simulink model "acc_integrated_model"  (R2024b)
settings: Solver=FixedStepDiscrete  StartTime=0.0  StopTime=inf  FixedStep=0.05  RelTol=1e-3
model workspace (MAT data in the model file):
  command_bp = [0 1 2 3 4 5 6 7]
  control_enabled_table = [1  1  1  1  1  1  0  0; 0  1  1  0  0  0  0  0; 0  1  0  0  0  0  0  0; 0  0  0  0  0  0  0  0]
  decision_raw_table = [-1  1  2  3  4  7  8  8; 8  5  6  8  8  8  8  8; 8  5  8  8  8  8  8  8; 8  8  8  8  8  8  8  8]
  decision_table = [-1  1  2  3  4  7  8  8; 8  5  6  8  8  8  8  8; 8  5  8  8  8  8  8  8; 8  8  8  8  8  8  8  8]
  next_state_table = [0  0  0  0  0  0  1  1; 1  0  0  1  1  1  1  1; 2  0  2  2  2  2  2  2; 3  3  3  3  3  3  3  3]
  side_effect_table = [0  0  0  0  0  0  0  0; 0  0  0  0  0  0  0  0; 0  1  0  0  0  0  0  0; 0  0  0  0  0  0  0  0]
  state_bp = [0 1 2 3]
undefined symbols (not defined in the file or in its folder): dspblkCoreblockFVToolHelper, f, gcbh
libraries: simulink x3, instrumentlib x2, sldvlib x1
settings Model: Creator=aiden  LastModifiedBy=aiden
settings DataIOCC: SaveOutput=off  SaveTime=off

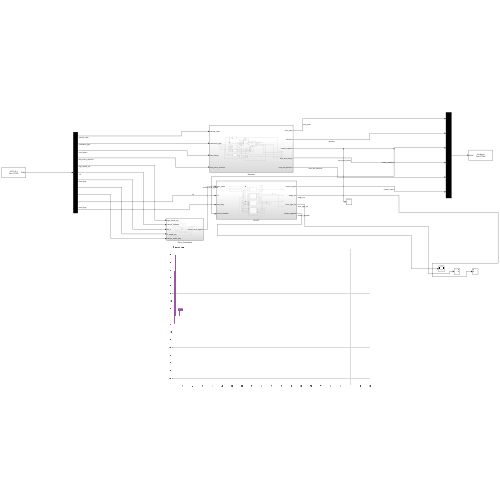
[thumbnail: Simulink's stored preview of the top-level diagram]
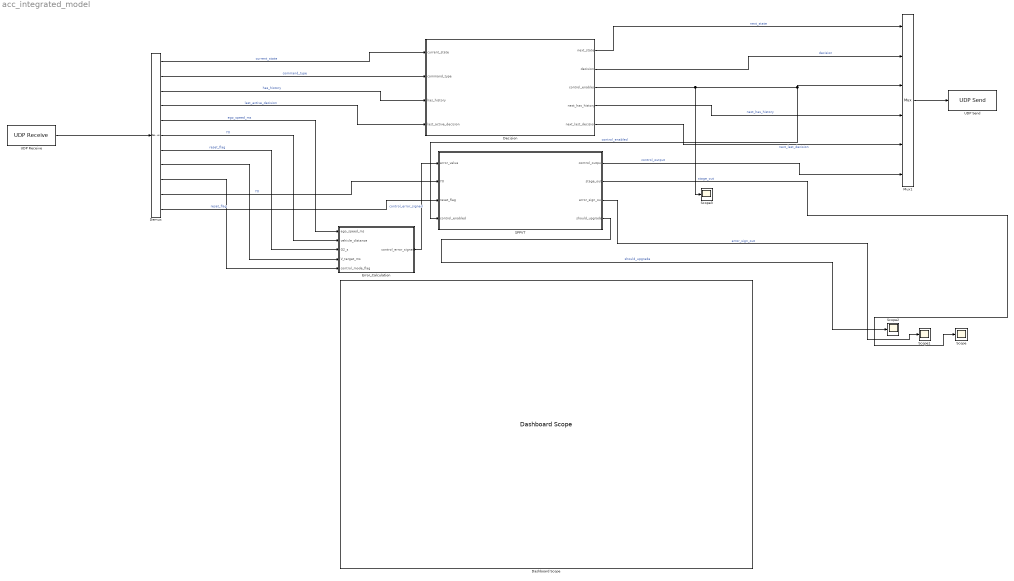
== system acc_integrated_model ==
  Dashboard Scope : DashboardScope  UpdateMode=Scroll
  Decision : Subsystem
  Demux : Demux  Outputs=11
  Error_Calculation : Subsystem
  Mux1 : Mux  Inputs=6
  SPPVT : Subsystem
  Scope{,1..3} (4 alike) : Scope
  UDP Receive : instrumentlib/UDP Receive  LocalAddress=127.0.0.1  LocalPort=27000  EnablePortSharing=off  Host=localhost  Port=9090  GetLatestData=on  DataSize=[ 11, 1 ]  DataType=double  ASCIIFormatting=%f,  Terminator=LF  CustomTerminator=10  ByteOrder=little-endian  EnableBlockingMode=on  Timeout=20  SampleTime=-1  SimulateUsing=Interpreted execution
  UDP Send : instrumentlib/UDP Send  Host=localhost  Port=27001  LocalAddress=0.0.0.0  LocalPort=27001  EnablePortSharing=on  OutputDatagramPacketSize=512  ByteOrder=little-endian  EnableBlockingMode=off  SimulateUsing=Interpreted execution
  wires:
  UDP Receive/1 -> Demux/1
  Demux/1 -> Decision/1(current_state)  "current_state"
  Demux/2 -> Decision/2(command_type)  "command_type"
  Demux/3 -> Decision/3(has_history)  "has_history"
  Demux/4 -> Decision/4(last_active_decision)  "last_active_decision"
  Error_Calculation/1(control_error_signed) -> SPPVT/1(error_value)  "control_error_signed"
  Demux/10 -> SPPVT/2(Y0)  "Y0"
  Demux/11 -> SPPVT/3(reset_flag)  "reset_flag"
  Decision/1(next_state) -> Mux1/1  "next_state"
  Decision/2(decision) -> Mux1/2  "decision"
  Decision/3(control_enabled) -> Scope3/1, Mux1/3, SPPVT/4(control_enabled)  "control_enabled"
  Decision/4(next_has_history) -> Mux1/4  "next_has_history"
  Decision/5(next_last_decision) -> Mux1/5  "next_last_decision"
  SPPVT/1(control_output) -> Mux1/6  "control_output"
  Mux1/1 -> UDP Send/1
  SPPVT/2(stage_out) -> Scope/1  "stage_out"
  SPPVT/3(error_sign_out) -> Scope1/1  "error_sign_out"
  SPPVT/4(should_upgrade) -> Scope2/1  "should_upgrade"
  Demux/5 -> Error_Calculation/1(ego_speed_ms)  "ego_speed_ms"
  Demux/6 -> Error_Calculation/2(vehicle_distance)  "Y0"
  Demux/7 -> Error_Calculation/3(G2_s)  "reset_flag"
  Demux/8 -> Error_Calculation/4(V_target_ms)
  Demux/9 -> Error_Calculation/5(control_mode_flag)

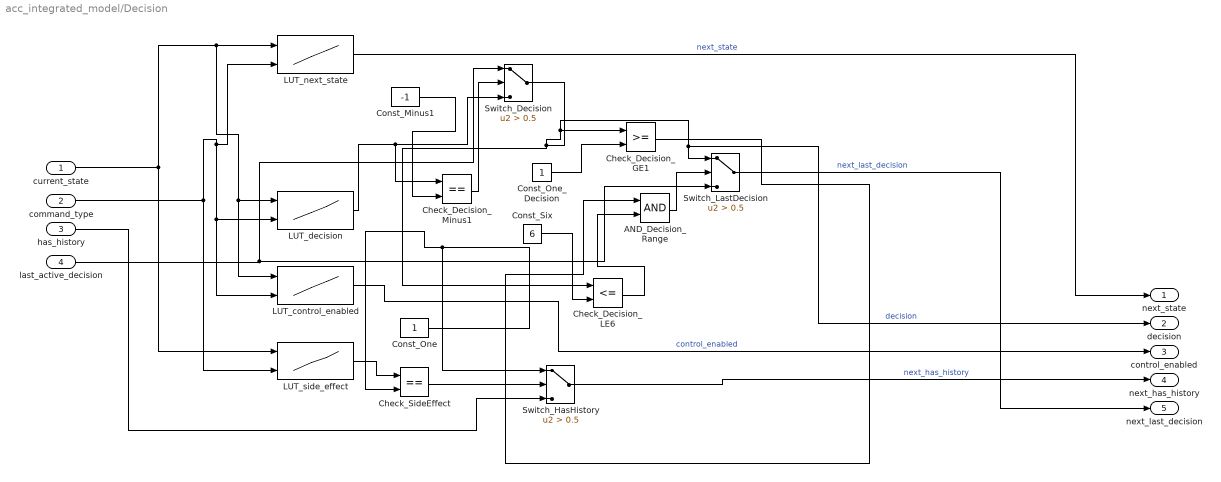
== system acc_integrated_model/Decision ==
  current_state : Inport
  command_type : Inport  Port=2
  has_history : Inport  Port=3
  last_active_decision : Inport  Port=4
  AND_Decision_Range : Logic  AllPortsSameDT=off  OutDataTypeStr=boolean
  Check_Decision_GE1 : RelationalOperator  OutDataTypeStr=boolean  RndMeth=Simplest  InputSameDT=off
  Check_Decision_LE6 : RelationalOperator  Operator=<=  OutDataTypeStr=boolean  RndMeth=Simplest  InputSameDT=off
  Check_Decision_Minus1 : RelationalOperator  Operator===  OutDataTypeStr=boolean  RndMeth=Simplest  InputSameDT=off
  Check_SideEffect : RelationalOperator  Operator===  OutDataTypeStr=boolean  RndMeth=Simplest  InputSameDT=off
  Const_Minus1 : Constant  Value=-1
  Const_One : Constant
  Const_One_Decision : Constant
  Const_Six : Constant  Value=6
  LUT_control_enabled : Lookup_n-D  BreakpointsForDimension1=state_bp  BreakpointsForDimension2=command_bp  BreakpointsForDimension3=[5, 7]  Table=control_enabled_table  InternalRulePriority=Speed  RndMeth=Simplest
      settings: InputPortMap=u0,u1
  LUT_decision : Lookup_n-D  BreakpointsForDimension1=state_bp  BreakpointsForDimension2=command_bp  BreakpointsForDimension3=[5, 7]  Table=decision_table  InternalRulePriority=Speed  RndMeth=Simplest
      settings: InputPortMap=u0,u1
  LUT_next_state : Lookup_n-D  BreakpointsForDimension1=state_bp  BreakpointsForDimension2=command_bp  BreakpointsForDimension3=[5, 7]  Table=next_state_table  InternalRulePriority=Speed  RndMeth=Simplest
      settings: InputPortMap=u0,u1
  LUT_side_effect : Lookup_n-D  BreakpointsForDimension1=state_bp  BreakpointsForDimension2=command_bp  BreakpointsForDimension3=[5, 7]  Table=side_effect_table  InternalRulePriority=Speed  RndMeth=Simplest
      settings: InputPortMap=u0,u1
  Switch_Decision : Switch  Criteria=u2 > Threshold  Threshold=0.5  SaturateOnIntegerOverflow=off  InputSameDT=off
  Switch_HasHistory : Switch  Criteria=u2 > Threshold  Threshold=0.5  SaturateOnIntegerOverflow=off  InputSameDT=off
  Switch_LastDecision : Switch  Criteria=u2 > Threshold  Threshold=0.5  SaturateOnIntegerOverflow=off  InputSameDT=off
  next_state : Outport
  decision : Outport  Port=2
  control_enabled : Outport  Port=3
  next_has_history : Outport  Port=4
  next_last_decision : Outport  Port=5
  wires:
  Check_Decision_GE1/1 -> AND_Decision_Range/1
  Check_Decision_LE6/1 -> AND_Decision_Range/2
  Const_Six/1 -> Check_Decision_LE6/2
  current_state/1 -> LUT_side_effect/1, LUT_decision/1, LUT_control_enabled/1, LUT_next_state/1
  last_active_decision/1 -> Switch_Decision/1, Switch_LastDecision/3
  Const_Minus1/1 -> Check_Decision_Minus1/2
  Switch_HasHistory/1 -> next_has_history/1  "next_has_history"
  AND_Decision_Range/1 -> Switch_LastDecision/2
  Check_Decision_Minus1/1 -> Switch_Decision/2
  Check_SideEffect/1 -> Switch_HasHistory/2
  LUT_control_enabled/1 -> control_enabled/1  "control_enabled"
  LUT_side_effect/1 -> Check_SideEffect/1
  Switch_Decision/1 -> decision/1, Switch_LastDecision/1, Check_Decision_GE1/1, Check_Decision_LE6/1  "decision"
  Const_One_Decision/1 -> Check_Decision_GE1/2
  command_type/1 -> LUT_side_effect/2, LUT_decision/2, LUT_control_enabled/2, LUT_next_state/2
  Switch_LastDecision/1 -> next_last_decision/1  "next_last_decision"
  has_history/1 -> Switch_HasHistory/3
  LUT_decision/1 -> Check_Decision_Minus1/1, Switch_Decision/3
  LUT_next_state/1 -> next_state/1  "next_state"
  Const_One/1 -> Check_SideEffect/2, Switch_HasHistory/1

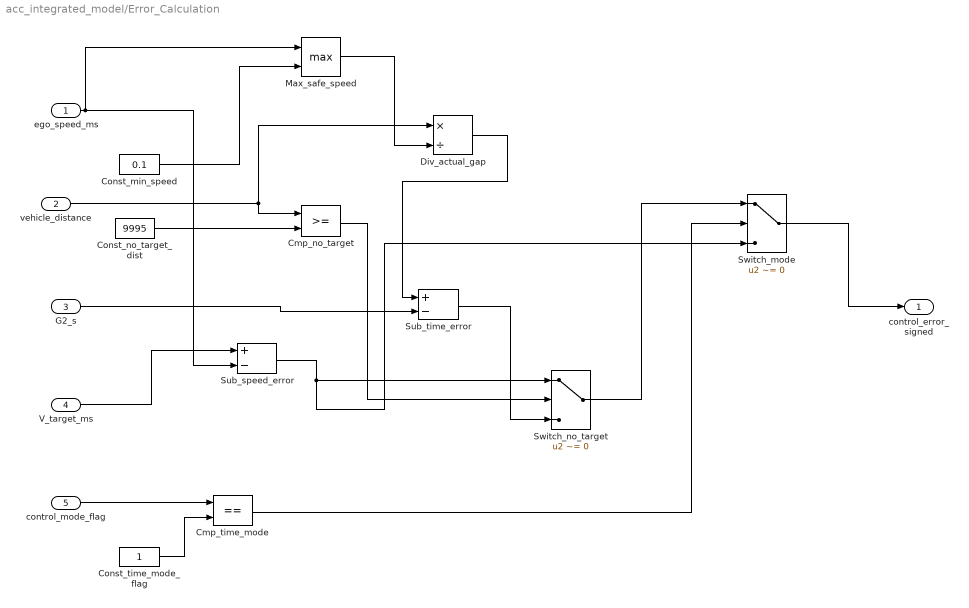
== system acc_integrated_model/Error_Calculation ==
  ego_speed_ms : Inport
  vehicle_distance : Inport  Port=2
  G2_s : Inport  Port=3
  V_target_ms : Inport  Port=4
  control_mode_flag : Inport  Port=5
  Cmp_no_target : RelationalOperator  OutDataTypeStr=boolean  RndMeth=Simplest  InputSameDT=off
  Cmp_time_mode : RelationalOperator  Operator===  OutDataTypeStr=boolean  RndMeth=Simplest  InputSameDT=off
  Const_min_speed : Constant  Value=0.1
  Const_no_target_dist : Constant  Value=9995
  Const_time_mode_flag : Constant
  Div_actual_gap : Product  Inputs=*/
  Max_safe_speed : MinMax  Function=max  Inputs=2
  Sub_speed_error : Sum  Inputs=+-
  Sub_time_error : Sum  Inputs=+-
  Switch_mode : Switch  Criteria=u2 ~= 0  SaturateOnIntegerOverflow=off  InputSameDT=off
  Switch_no_target : Switch  Criteria=u2 ~= 0  SaturateOnIntegerOverflow=off  InputSameDT=off
  control_error_signed : Outport
  wires:
  V_target_ms/1 -> Sub_speed_error/1
  ego_speed_ms/1 -> Sub_speed_error/2, Max_safe_speed/1
  Const_min_speed/1 -> Max_safe_speed/2
  vehicle_distance/1 -> Div_actual_gap/1, Cmp_no_target/1
  Max_safe_speed/1 -> Div_actual_gap/2
  Div_actual_gap/1 -> Sub_time_error/1
  G2_s/1 -> Sub_time_error/2
  Const_no_target_dist/1 -> Cmp_no_target/2
  Sub_speed_error/1 -> Switch_mode/3, Switch_no_target/1
  Cmp_no_target/1 -> Switch_no_target/2
  Sub_time_error/1 -> Switch_no_target/3
  control_mode_flag/1 -> Cmp_time_mode/1
  Const_time_mode_flag/1 -> Cmp_time_mode/2
  Switch_no_target/1 -> Switch_mode/1
  Cmp_time_mode/1 -> Switch_mode/2
  Switch_mode/1 -> control_error_signed/1

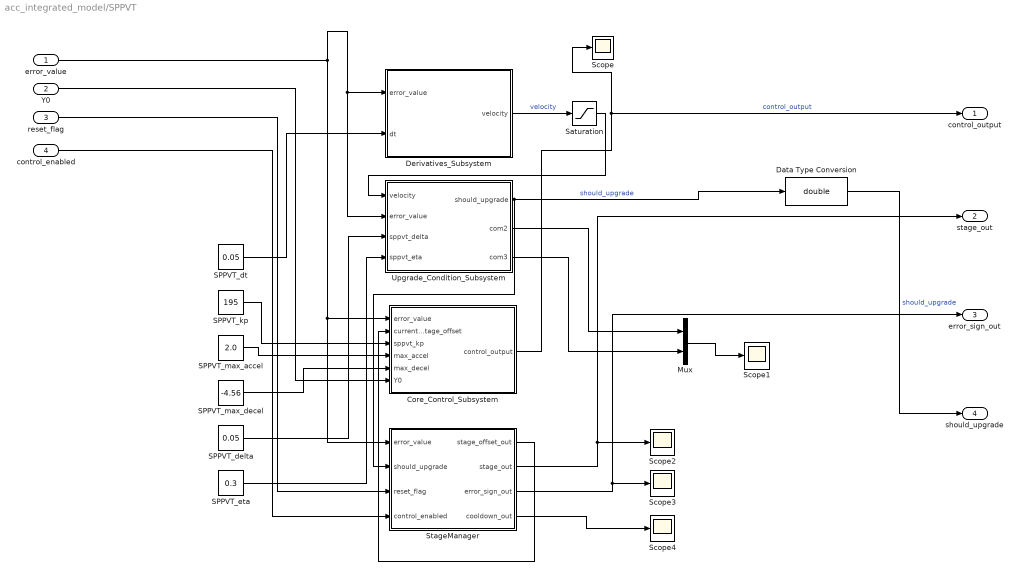
== system acc_integrated_model/SPPVT ==
  error_value : Inport
  Y0 : Inport  Port=2
  reset_flag : Inport  Port=3
  control_enabled : Inport  Port=4
  Core_Control_Subsystem : Subsystem
  Data Type Conversion : DataTypeConversion  OutDataTypeStr=double  SaturateOnIntegerOverflow=off  RndMeth=Floor
  Derivatives_Subsystem : Subsystem
  Mux : Mux  Inputs=2
  SPPVT_delta : Constant  Value=0.05
  SPPVT_dt : Constant  Value=0.05
  SPPVT_eta : Constant  Value=0.3
  SPPVT_kp : Constant  Value=195
  SPPVT_max_accel : Constant  Value=2.0
  SPPVT_max_decel : Constant  Value=-4.56
  Saturation : Saturate  UpperLimit=5000.0  LowerLimit=-5000.0
  Scope{,1..4} (5 alike) : Scope
  StageManager : Subsystem
  Upgrade_Condition_Subsystem : Subsystem
  control_output : Outport
  stage_out : Outport  Port=2
  error_sign_out : Outport  Port=3
  should_upgrade : Outport  Port=4
  wires:
  SPPVT_kp/1 -> Core_Control_Subsystem/3(sppvt_kp)
  Derivatives_Subsystem/1(velocity) -> Saturation/1  "velocity"
  Core_Control_Subsystem/1(control_output) -> Scope/1, control_output/1  "control_output"
  Data Type Conversion/1 -> should_upgrade/1  "should_upgrade"
  Saturation/1 -> Upgrade_Condition_Subsystem/1(velocity)
  SPPVT_max_accel/1 -> Core_Control_Subsystem/4(max_accel)
  Upgrade_Condition_Subsystem/1(should_upgrade) -> StageManager/2(should_upgrade), Data Type Conversion/1  "should_upgrade"
  SPPVT_dt/1 -> Derivatives_Subsystem/2(dt)
  Upgrade_Condition_Subsystem/2(com2) -> Mux/1
  SPPVT_eta/1 -> Upgrade_Condition_Subsystem/4(sppvt_eta)
  SPPVT_delta/1 -> Upgrade_Condition_Subsystem/3(sppvt_delta)
  error_value/1 -> Core_Control_Subsystem/1(error_value), StageManager/1(error_value), Upgrade_Condition_Subsystem/2(error_value), Derivatives_Subsystem/1(error_value)
  Mux/1 -> Scope1/1
  SPPVT_max_decel/1 -> Core_Control_Subsystem/5(max_decel)
  Upgrade_Condition_Subsystem/3(com3) -> Mux/2
  reset_flag/1 -> StageManager/3(reset_flag)
  control_enabled/1 -> StageManager/4(control_enabled)
  StageManager/1(stage_offset_out) -> Core_Control_Subsystem/2(current_stage_offset)
  StageManager/2(stage_out) -> stage_out/1, Scope2/1
  StageManager/3(error_sign_out) -> error_sign_out/1, Scope3/1
  StageManager/4(cooldown_out) -> Scope4/1
  Y0/1 -> Core_Control_Subsystem/6(Y0)

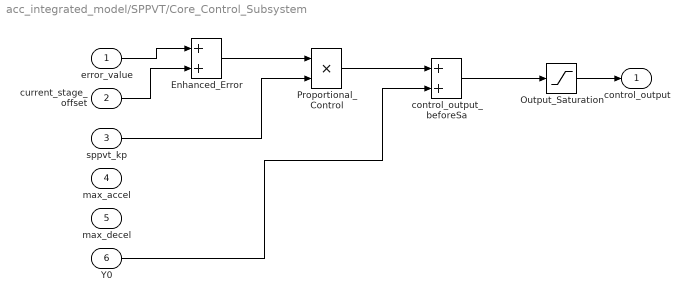
== system acc_integrated_model/SPPVT/Core_Control_Subsystem ==
  error_value : Inport
  current_stage_offset : Inport  Port=2
  sppvt_kp : Inport  Port=3
  max_accel : Inport  Port=4
  max_decel : Inport  Port=5
  Y0 : Inport  Port=6
  Enhanced_Error : Sum
  Output_Saturation : Saturate  UpperLimit=800  LowerLimit=-800
  Proportional_Control : Product
  control_output_beforeSa : Sum
  control_output : Outport
  wires:
  Proportional_Control/1 -> control_output_beforeSa/1
  Output_Saturation/1 -> control_output/1
  sppvt_kp/1 -> Proportional_Control/2
  current_stage_offset/1 -> Enhanced_Error/2
  error_value/1 -> Enhanced_Error/1
  Enhanced_Error/1 -> Proportional_Control/1
  Y0/1 -> control_output_beforeSa/2
  control_output_beforeSa/1 -> Output_Saturation/1

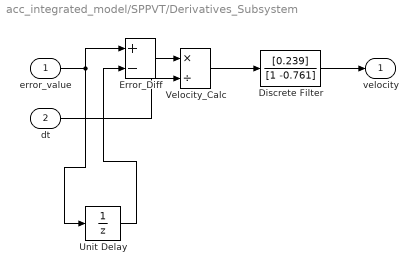
== system acc_integrated_model/SPPVT/Derivatives_Subsystem ==
  error_value : Inport
  dt : Inport  Port=2
  Discrete Filter : DiscreteFilter  LoadFcn=dspblkCoreblockFVToolHelper(gcbh,'load');  Numerator=[0.239]  Denominator=[1 -0.761]
      settings: CopyFcn=dspblkCoreblockFVToolHelper(gcbh,'copy');  DeleteFcn=dspblkCoreblockFVToolHelper(gcbh,'close');  ModelCloseFcn=dspblkCoreblockFVToolHelper(gcbh,'close');  PreSaveFcn=dspblkCoreblockFVToolHelper(gcbh,'presave');  PostSaveFcn=dspblkCoreblockFVToolHelper(gcbh,'postsave');  CloseFcn=dspblkCoreblockFVToolHelper(gcbh,'close');
  Error_Diff : Sum  Inputs=+-
  Unit Delay : UnitDelay  SampleTime=-1  HasFrameUpgradeWarning=on
  Velocity_Calc : Product  Inputs=*/
  velocity : Outport
  wires:
  Velocity_Calc/1 -> Discrete Filter/1
  error_value/1 -> Unit Delay/1, Error_Diff/1
  Error_Diff/1 -> Velocity_Calc/1
  dt/1 -> Velocity_Calc/2
  Discrete Filter/1 -> velocity/1
  Unit Delay/1 -> Error_Diff/2

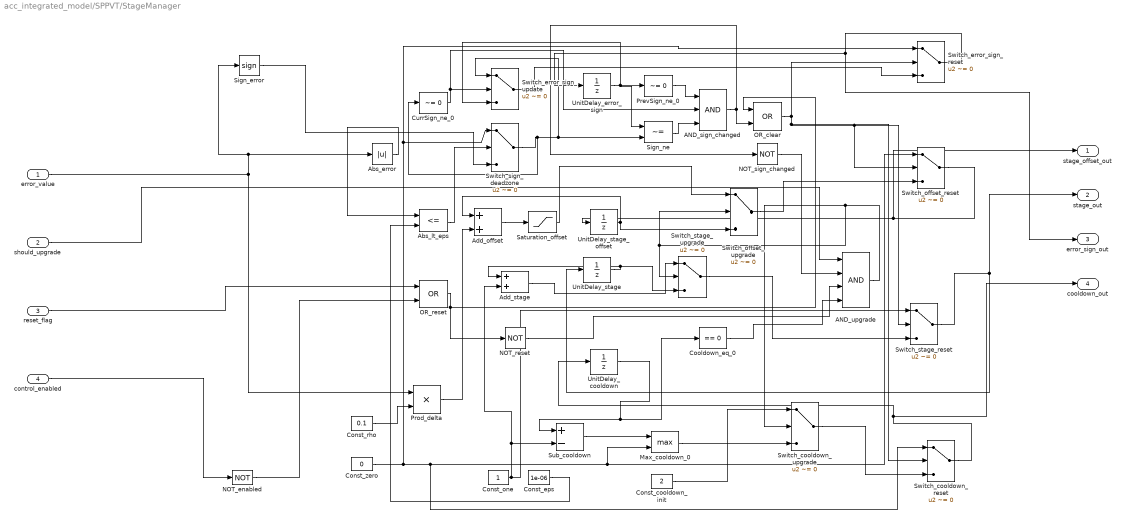
== system acc_integrated_model/SPPVT/StageManager ==
  error_value : Inport
  should_upgrade : Inport  Port=2
  reset_flag : Inport  Port=3
  control_enabled : Inport  Port=4
  AND_sign_changed : Logic  Inputs=3  AllPortsSameDT=off  OutDataTypeStr=boolean
  AND_upgrade : Logic  Inputs=4  AllPortsSameDT=off  OutDataTypeStr=boolean
  Abs_error : Abs  SaturateOnIntegerOverflow=off
  Abs_lt_eps : RelationalOperator  Operator=<=  OutDataTypeStr=boolean  RndMeth=Simplest  InputSameDT=off
  Add_offset : Sum
  Add_stage : Sum
  Const_cooldown_init : Constant  Value=2
  Const_eps : Constant  Value=1e-06
  Const_one : Constant
  Const_rho : Constant  Value=0.1
  Const_zero : Constant  Value=0
  Cooldown_eq_0 : simulink/Logic and Bit Operations/Compare To Zero  relop===  OutDataTypeStr=boolean
  CurrSign_ne_0 : simulink/Logic and Bit Operations/Compare To Zero  relop=~=  OutDataTypeStr=boolean
  Max_cooldown_0 : MinMax  Function=max  Inputs=2
  NOT_enabled : Logic  Operator=NOT  AllPortsSameDT=off  OutDataTypeStr=boolean
  NOT_reset : Logic  Operator=NOT  AllPortsSameDT=off  OutDataTypeStr=boolean
  NOT_sign_changed : Logic  Operator=NOT  AllPortsSameDT=off  OutDataTypeStr=boolean
  OR_clear : Logic  Operator=OR  AllPortsSameDT=off  OutDataTypeStr=boolean
  OR_reset : Logic  Operator=OR  AllPortsSameDT=off  OutDataTypeStr=boolean
  PrevSign_ne_0 : simulink/Logic and Bit Operations/Compare To Zero  relop=~=  OutDataTypeStr=boolean
  Prod_delta : Product
  Saturation_offset : Saturate  UpperLimit=500  LowerLimit=-500
  Sign_error : Signum
  Sign_ne : RelationalOperator  Operator=~=  OutDataTypeStr=boolean  RndMeth=Simplest  InputSameDT=off
  Sub_cooldown : Sum  Inputs=+-
  Switch_cooldown_reset : Switch  Criteria=u2 ~= 0  SaturateOnIntegerOverflow=off  InputSameDT=off
  Switch_cooldown_upgrade : Switch  Criteria=u2 ~= 0  SaturateOnIntegerOverflow=off  InputSameDT=off
  Switch_error_sign_reset : Switch  Criteria=u2 ~= 0  SaturateOnIntegerOverflow=off  InputSameDT=off
  Switch_error_sign_update : Switch  Criteria=u2 ~= 0  SaturateOnIntegerOverflow=off  InputSameDT=off
  Switch_offset_reset : Switch  Criteria=u2 ~= 0  SaturateOnIntegerOverflow=off  InputSameDT=off
  Switch_offset_upgrade : Switch  Criteria=u2 ~= 0  SaturateOnIntegerOverflow=off  InputSameDT=off
  Switch_sign_deadzone : Switch  Criteria=u2 ~= 0  SaturateOnIntegerOverflow=off  InputSameDT=off
  Switch_stage_reset : Switch  Criteria=u2 ~= 0  SaturateOnIntegerOverflow=off  InputSameDT=off
  Switch_stage_upgrade : Switch  Criteria=u2 ~= 0  SaturateOnIntegerOverflow=off  InputSameDT=off
  UnitDelay_cooldown : UnitDelay  SampleTime=-1  HasFrameUpgradeWarning=on
  UnitDelay_error_sign : UnitDelay  SampleTime=-1  HasFrameUpgradeWarning=on
  UnitDelay_stage : UnitDelay  InitialCondition=1  SampleTime=-1  HasFrameUpgradeWarning=on
  UnitDelay_stage_offset : UnitDelay  SampleTime=-1  HasFrameUpgradeWarning=on
  stage_offset_out : Outport
  stage_out : Outport  Port=2
  error_sign_out : Outport  Port=3
  cooldown_out : Outport  Port=4
  wires:
  control_enabled/1 -> NOT_enabled/1
  reset_flag/1 -> OR_reset/1
  NOT_enabled/1 -> OR_reset/2
  error_value/1 -> Sign_error/1, Abs_error/1, Prod_delta/1
  Abs_error/1 -> Abs_lt_eps/1
  Const_eps/1 -> Abs_lt_eps/2
  Const_zero/1 -> Switch_sign_deadzone/1, Switch_error_sign_reset/1, Switch_offset_reset/1, Max_cooldown_0/2, Switch_cooldown_reset/1
  Abs_lt_eps/1 -> Switch_sign_deadzone/2
  Sign_error/1 -> Switch_sign_deadzone/3
  Switch_sign_deadzone/1 -> Sign_ne/2, Switch_error_sign_update/1, CurrSign_ne_0/1
  UnitDelay_error_sign/1 -> PrevSign_ne_0/1, Sign_ne/1, Switch_error_sign_update/3
  PrevSign_ne_0/1 -> AND_sign_changed/1
  CurrSign_ne_0/1 -> AND_sign_changed/2, Switch_error_sign_update/2
  Sign_ne/1 -> AND_sign_changed/3
  OR_reset/1 -> OR_clear/1, NOT_reset/1
  AND_sign_changed/1 -> OR_clear/2, NOT_sign_changed/1
  should_upgrade/1 -> AND_upgrade/1
  NOT_sign_changed/1 -> AND_upgrade/2
  NOT_reset/1 -> AND_upgrade/3
  UnitDelay_cooldown/1 -> Cooldown_eq_0/1, Sub_cooldown/1
  Cooldown_eq_0/1 -> AND_upgrade/4
  Const_rho/1 -> Prod_delta/2
  UnitDelay_stage_offset/1 -> Add_offset/1, Switch_offset_upgrade/3
  Prod_delta/1 -> Add_offset/2
  Add_offset/1 -> Saturation_offset/1
  Saturation_offset/1 -> Switch_offset_upgrade/1
  AND_upgrade/1 -> Switch_offset_upgrade/2, Switch_stage_upgrade/2, Switch_cooldown_upgrade/2
  OR_clear/1 -> Switch_offset_reset/2, Switch_stage_reset/2, Switch_cooldown_reset/2, Switch_error_sign_reset/2
  Switch_offset_upgrade/1 -> Switch_offset_reset/3
  Switch_offset_reset/1 -> UnitDelay_stage_offset/1, stage_offset_out/1
  Switch_error_sign_update/1 -> Switch_error_sign_reset/3
  Switch_error_sign_reset/1 -> error_sign_out/1, UnitDelay_error_sign/1
  Const_one/1 -> Sub_cooldown/2, Add_stage/2, Switch_stage_reset/1
  Sub_cooldown/1 -> Max_cooldown_0/1
  Const_cooldown_init/1 -> Switch_cooldown_upgrade/1
  Max_cooldown_0/1 -> Switch_cooldown_upgrade/3
  Switch_cooldown_upgrade/1 -> Switch_cooldown_reset/3
  Switch_cooldown_reset/1 -> UnitDelay_cooldown/1, cooldown_out/1
  UnitDelay_stage/1 -> Add_stage/1, Switch_stage_upgrade/3
  Add_stage/1 -> Switch_stage_upgrade/1
  Switch_stage_upgrade/1 -> Switch_stage_reset/3
  Switch_stage_reset/1 -> UnitDelay_stage/1, stage_out/1

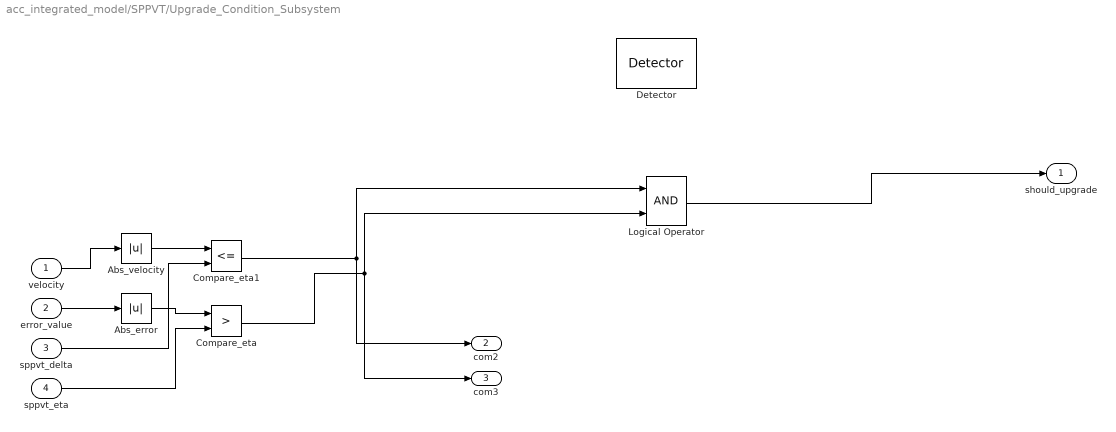
== system acc_integrated_model/SPPVT/Upgrade_Condition_Subsystem ==
  velocity : Inport
  error_value : Inport  Port=2
  sppvt_delta : Inport  Port=3
  sppvt_eta : Inport  Port=4
  Abs_error : Abs  SaturateOnIntegerOverflow=off
  Abs_velocity : Abs  SaturateOnIntegerOverflow=off
  Compare_eta : RelationalOperator  Operator=>  OutDataTypeStr=boolean  RndMeth=Simplest  InputSameDT=off
  Compare_eta1 : RelationalOperator  Operator=<=  OutDataTypeStr=boolean  RndMeth=Simplest  InputSameDT=off
  Detector : sldvlib/Temporal Operators/Detector  reset=off  typ=Delayed Fixed Duration  in_hold=4  delay=1  out_hold=1
  Logical Operator : Logic  AllPortsSameDT=off  OutDataTypeStr=boolean
  should_upgrade : Outport
  com2 : Outport  Port=2
  com3 : Outport  Port=3
  wires:
  error_value/1 -> Abs_error/1
  Abs_error/1 -> Compare_eta/1
  sppvt_eta/1 -> Compare_eta/2
  velocity/1 -> Abs_velocity/1
  Abs_velocity/1 -> Compare_eta1/1
  sppvt_delta/1 -> Compare_eta1/2
  Compare_eta1/1 -> com2/1, Logical Operator/1
  Compare_eta/1 -> Logical Operator/2, com3/1
  Logical Operator/1 -> should_upgrade/1
